simulink model "Racing_2019"  (R2017a)
settings: Solver=FixedStepDiscrete  StartTime=0.0  StopTime=Inf  FixedStep=1e-3  RelTol=1e-3  EnableMultiTasking=on
PostLoadFcn:
  | , if any(exist('dsrtsu_mdlpostloadfcn', 'file') == [2, 3, 6]), try dsrtsu_mdlpostloadfcn('Execute', bdroot); catch fprintf('Error in PostLoadFcn (dsrtsu_mdlpostloadfcn) for model "%s":\n %s\n', bdroot, lasterr); end, end,
undefined symbols (not defined in the file): Accu_Fans_Enable, Accu_Fans_ON, Accu_Fans_PWM, APPS_Bypass, APPS_Value, AUX_Error_Time, Batt_Temp_High_Threshold, Batt_Temp_Low_Threshold, BMS_Error_Time, BMS_Reset, BMS_Reset_Enable, BMS_Status_Bypass, Brake_Plausibility_Threshold, Brake_Threshold, Brakelight_Test, Braking_Torque, BSPD_State_Bypass, Buzzer, Buzzer_Silent, Buzzer_Test, Calibrate, CAN_Rx_FMEA_Enable, CAN_Status_FMEA_Enable, CAN_Tx_FMEA_Enable, Car_Reset, Car_Reset_Enable, Dash_Fan_PWM, DiscIntNeverNeededParam, DRS_Enable, DRS_PWM_OFF, DRS_PWM_ON, ED_Enable, ED_On, Eject_USB, Enable_Kill, Enable_LED_Test, Fans_Left_Enable, Fans_Left_ON, Fans_Left_PWM, Fans_Right_Enable, Fans_Right_ON, Fans_Right_PWM, I_MAX, IGBT_Temp_High_Threshold, IGBT_Temp_Low_Threshold, Inverter_CAN_Tx_Enable, Inverter_Frequency, KW_Max_Regen_Reset, KW_Max_Reset, LV_DCDC_Temp_High_Threshold, LV_DCDC_Temp_Low_Threshold, magnitude, Plausibility_Bypass, Power_Limiter_Killswitch, Power_Target_kW, Pump_Left_Enable, Pump_Left_ON, Pump_Right_Enable, Pump_Right_ON, Pump_Signal_Left ... (+13)
libraries: rtiusbflightreclib x206, simulink x153, rtican x52, powerlib_meascontrol x47, simulink_extras x17, rti1401lib_adc_type4 x6, rti1401lib_dio_type4 x3, rti1401lib_II_base x1
(part 22 of 23)

== system Racing_2019/CAN Configuration/Accu CAN Rx ==
  Rx Messages : Inport
  Accu Baudrate Rx : Memory  InheritSampleTime=on
  Compare To Constant : simulink/Logic and Bit Operations/Compare To Constant  relop=>=  const=999  OutDataTypeStr=boolean
  Counter Limited : simulink/Sources/Counter Limited  uplimit=1000  tsamp=0.001
  Delay 2ms : Delay
  Memory1 : Memory  InheritSampleTime=on
  Moving Baudrate : Sum  Inputs=+-
  Switch : Switch  Criteria=u2 > Threshold
  Switch1 : Switch  Criteria=u2 > Threshold
  "Rx Baudrate " : Outport
  wires:
  Switch/1 -> Memory1/1
  Memory1/1 -> Moving Baudrate/2, Switch/3
  Counter Limited/1 -> Compare To Constant/1
  Switch1/1 -> Accu Baudrate Rx/1
  Compare To Constant/1 -> Delay 2ms/1, Switch1/2
  Accu Baudrate Rx/1 -> "Rx Baudrate "/1, Switch1/3
  Delay 2ms/1 -> Switch/2
  Rx Messages/1 -> Moving Baudrate/1, Switch/1
  Moving Baudrate/1 -> Switch1/1

== system Racing_2019/CAN Configuration/Accu CAN Tx ==
  Tx Messages : Inport
  Accu Baudrate Tx : Memory  InheritSampleTime=on
  Compare To Constant : simulink/Logic and Bit Operations/Compare To Constant  relop=>=  const=999  OutDataTypeStr=boolean
  Counter Limited : simulink/Sources/Counter Limited  uplimit=1000  tsamp=0.001
  Delay 2ms : Delay
  Memory1 : Memory  InheritSampleTime=on
  Moving Baudrate : Sum  Inputs=+-
  Switch : Switch  Criteria=u2 > Threshold
  Switch1 : Switch  Criteria=u2 > Threshold
  "Tx Baudrate " : Outport
  wires:
  Switch/1 -> Memory1/1
  Memory1/1 -> Moving Baudrate/2, Switch/3
  Counter Limited/1 -> Compare To Constant/1
  Switch1/1 -> Accu Baudrate Tx/1
  Compare To Constant/1 -> Delay 2ms/1, Switch1/2
  Accu Baudrate Tx/1 -> "Tx Baudrate "/1, Switch1/3
  Delay 2ms/1 -> Switch/2
  Tx Messages/1 -> Moving Baudrate/1, Switch/1
  Moving Baudrate/1 -> Switch1/1

== system Racing_2019/CAN Configuration/Dash-Aux CAN Rx ==
  Rx Messages : Inport
  Compare To Constant : simulink/Logic and Bit Operations/Compare To Constant  relop=>=  const=999  OutDataTypeStr=boolean
  Counter Limited : simulink/Sources/Counter Limited  uplimit=1000  tsamp=0.001
  Dash-Aux Baudrate Rx : Memory  InheritSampleTime=on
  Delay 2ms : Delay
  Memory1 : Memory  InheritSampleTime=on
  Moving Baudrate : Sum  Inputs=+-
  Switch : Switch  Criteria=u2 > Threshold
  Switch1 : Switch  Criteria=u2 > Threshold
  Rx Baudrate : Outport
  wires:
  Switch/1 -> Memory1/1
  Memory1/1 -> Moving Baudrate/2, Switch/3
  Counter Limited/1 -> Compare To Constant/1
  Switch1/1 -> Dash-Aux Baudrate Rx/1
  Compare To Constant/1 -> Delay 2ms/1, Switch1/2
  Dash-Aux Baudrate Rx/1 -> Rx Baudrate/1, Switch1/3
  Delay 2ms/1 -> Switch/2
  Rx Messages/1 -> Moving Baudrate/1, Switch/1
  Moving Baudrate/1 -> Switch1/1

== system Racing_2019/CAN Configuration/Dash-Aux CAN Tx ==
  Tx Messages : Inport
  Compare To Constant : simulink/Logic and Bit Operations/Compare To Constant  relop=>=  const=999  OutDataTypeStr=boolean
  Counter Limited : simulink/Sources/Counter Limited  uplimit=1000  tsamp=0.001
  Dash-Aux Baudrate Tx : Memory  InheritSampleTime=on
  Delay 2ms : Delay
  Memory1 : Memory  InheritSampleTime=on
  Moving Baudrate : Sum  Inputs=+-
  Switch : Switch  Criteria=u2 > Threshold
  Switch1 : Switch  Criteria=u2 > Threshold
  Tx Baudrate : Outport
  wires:
  Switch/1 -> Memory1/1
  Memory1/1 -> Moving Baudrate/2, Switch/3
  Counter Limited/1 -> Compare To Constant/1
  Switch1/1 -> Dash-Aux Baudrate Tx/1
  Compare To Constant/1 -> Delay 2ms/1, Switch1/2
  Dash-Aux Baudrate Tx/1 -> Tx Baudrate/1, Switch1/3
  Delay 2ms/1 -> Switch/2
  Tx Messages/1 -> Moving Baudrate/1, Switch/1
  Moving Baudrate/1 -> Switch1/1

== system Racing_2019/CAN Configuration/Inverter LEFT CAN Rx ==
  Rx Messages : Inport
  Compare To Constant : simulink/Logic and Bit Operations/Compare To Constant  relop=>=  const=999  OutDataTypeStr=boolean
  Counter Limited : simulink/Sources/Counter Limited  uplimit=1000  tsamp=0.001
  Delay 2ms : Delay
  Inverter LEFT Baudrate Rx : Memory  InheritSampleTime=on
  Memory1 : Memory  InheritSampleTime=on
  Moving Baudrate : Sum  Inputs=+-
  Switch : Switch  Criteria=u2 > Threshold
  Switch1 : Switch  Criteria=u2 > Threshold
  "Rx Baudrate " : Outport
  wires:
  Switch/1 -> Memory1/1
  Memory1/1 -> Moving Baudrate/2, Switch/3
  Counter Limited/1 -> Compare To Constant/1
  Switch1/1 -> Inverter LEFT Baudrate Rx/1
  Compare To Constant/1 -> Delay 2ms/1, Switch1/2
  Inverter LEFT Baudrate Rx/1 -> "Rx Baudrate "/1, Switch1/3
  Delay 2ms/1 -> Switch/2
  Rx Messages/1 -> Moving Baudrate/1, Switch/1
  Moving Baudrate/1 -> Switch1/1

== system Racing_2019/CAN Configuration/Inverter LEFT CAN Tx ==
  Tx Messages : Inport
  Compare To Constant : simulink/Logic and Bit Operations/Compare To Constant  relop=>=  const=999  OutDataTypeStr=boolean
  Counter Limited : simulink/Sources/Counter Limited  uplimit=1000  tsamp=0.001
  Delay 2ms : Delay
  Inverter LEFT Baudrate Tx : Memory  InheritSampleTime=on
  Memory1 : Memory  InheritSampleTime=on
  Moving Baudrate : Sum  Inputs=+-
  Switch : Switch  Criteria=u2 > Threshold
  Switch1 : Switch  Criteria=u2 > Threshold
  Tx Baudrate : Outport
  wires:
  Switch/1 -> Memory1/1
  Memory1/1 -> Moving Baudrate/2, Switch/3
  Counter Limited/1 -> Compare To Constant/1
  Switch1/1 -> Inverter LEFT Baudrate Tx/1
  Compare To Constant/1 -> Delay 2ms/1, Switch1/2
  Inverter LEFT Baudrate Tx/1 -> Tx Baudrate/1, Switch1/3
  Delay 2ms/1 -> Switch/2
  Tx Messages/1 -> Moving Baudrate/1, Switch/1
  Moving Baudrate/1 -> Switch1/1

== system Racing_2019/CAN Configuration/Inverter RIGHT CAN Rx ==
  Rx Messages : Inport
  Compare To Constant : simulink/Logic and Bit Operations/Compare To Constant  relop=>=  const=999  OutDataTypeStr=boolean
  Counter Limited : simulink/Sources/Counter Limited  uplimit=1000  tsamp=0.001
  Delay 1ms : Delay  DelayLength=1
  Inverter RIGHT Baudrate Rx : Memory  InheritSampleTime=on
  Memory1 : Memory  InheritSampleTime=on
  Moving Baudrate : Sum  Inputs=+-
  Switch : Switch  Criteria=u2 > Threshold
  Switch1 : Switch  Criteria=u2 > Threshold
  "Rx Baudrate " : Outport
  wires:
  Switch/1 -> Memory1/1
  Memory1/1 -> Moving Baudrate/2, Switch/3
  Counter Limited/1 -> Compare To Constant/1
  Switch1/1 -> Inverter RIGHT Baudrate Rx/1
  Compare To Constant/1 -> Delay 1ms/1, Switch1/2
  Inverter RIGHT Baudrate Rx/1 -> "Rx Baudrate "/1, Switch1/3
  Delay 1ms/1 -> Switch/2
  Rx Messages/1 -> Moving Baudrate/1, Switch/1
  Moving Baudrate/1 -> Switch1/1

== system Racing_2019/CAN Configuration/Inverter RIGHT CAN Tx ==
  Tx Messages : Inport
  Compare To Constant : simulink/Logic and Bit Operations/Compare To Constant  relop=>=  const=999  OutDataTypeStr=boolean
  Counter Limited : simulink/Sources/Counter Limited  uplimit=1000  tsamp=0.001
  Delay 1ms : Delay  DelayLength=1
  Inverter LEFT Baudrate Tx : Memory  InheritSampleTime=on
  Memory1 : Memory  InheritSampleTime=on
  Moving Baudrate : Sum  Inputs=+-
  Switch : Switch  Criteria=u2 > Threshold
  Switch1 : Switch  Criteria=u2 > Threshold
  "Tx Baudrate " : Outport
  wires:
  Switch/1 -> Memory1/1
  Memory1/1 -> Moving Baudrate/2, Switch/3
  Counter Limited/1 -> Compare To Constant/1
  Switch1/1 -> Inverter LEFT Baudrate Tx/1
  Compare To Constant/1 -> Delay 1ms/1, Switch1/2
  Inverter LEFT Baudrate Tx/1 -> "Tx Baudrate "/1, Switch1/3
  Delay 1ms/1 -> Switch/2
  Tx Messages/1 -> Moving Baudrate/1, Switch/1
  Moving Baudrate/1 -> Switch1/1

== system Racing_2019/General Inputs/Dynamic Offset LEM IAC Left  ==
  Value : Inport
  Add : Sum
  Average Offset LEM Left : Product  Inputs=*/
  Compare To Constant : simulink/Logic and Bit Operations/Compare To Constant  relop=>=  const=10000  OutDataTypeStr=boolean
  Compare To Constant1 : simulink/Logic and Bit Operations/Compare To Constant  relop=<=  const=10001  OutDataTypeStr=boolean
  Constant : Constant  Value=0
  Constant1 : Constant  Value=Calibrate
  Constant2 : Constant  Value=0
  Counter Free-Running : simulink/Sources/Counter Free-Running  NumBits=14  tsamp=-1
  Delay : Delay  DelayLength=1
  Dynamic Offset LEM Left : Memory  InheritSampleTime=on
  Logical Operator : Logic  Operator=OR  AllPortsSameDT=off  OutDataTypeStr=boolean
  Logical Operator1 : Logic  Operator=NOT  AllPortsSameDT=off  OutDataTypeStr=boolean
  Logical Operator2 : Logic  AllPortsSameDT=off  OutDataTypeStr=boolean
  Memory LEM IAC Left : Memory
  S-R Flip-Flop LEM Left : simulink_extras/Flip Flops/S-R Flip-Flop  initial_condition=0
  Switch : Switch  Criteria=u2 > Threshold
  Switch1 : Switch  Criteria=u2 > Threshold
  Terminator : Terminator
  LEM IAC Left Dynamic Offset : Outport
  wires:
  Counter Free-Running/1 -> Compare To Constant/1, Average Offset LEM Left/2, Compare To Constant1/1
  Switch/1 -> Dynamic Offset LEM Left/1
  Memory LEM IAC Left/1 -> Average Offset LEM Left/1, Add/1
  Dynamic Offset LEM Left/1 -> LEM IAC Left Dynamic Offset/1, Switch/1
  Value/1 -> Add/2
  Average Offset LEM Left/1 -> Switch/3
  S-R Flip-Flop LEM Left/1 -> Switch/2
  S-R Flip-Flop LEM Left/2 -> Terminator/1
  Constant/1 -> Logical Operator/1
  Logical Operator/1 -> S-R Flip-Flop LEM Left/2
  Constant1/1 -> Logical Operator/2
  Switch1/1 -> Memory LEM IAC Left/1
  Add/1 -> Switch1/1
  Constant2/1 -> Switch1/3
  Logical Operator1/1 -> Delay/1
  Delay/1 -> Switch1/2
  Logical Operator2/1 -> S-R Flip-Flop LEM Left/1
  Compare To Constant/1 -> Logical Operator1/1, Logical Operator2/1
  Compare To Constant1/1 -> Logical Operator2/2

== system Racing_2019/General Inputs/Dynamic Offset LEM IAC Right ==
  Value : Inport
  Add : Sum
  Average Offset LEM Right : Product  Inputs=*/
  Compare To Constant : simulink/Logic and Bit Operations/Compare To Constant  relop=>=  const=10000  OutDataTypeStr=boolean
  Compare To Constant1 : simulink/Logic and Bit Operations/Compare To Constant  relop=<=  const=10001  OutDataTypeStr=boolean
  Constant : Constant  Value=0
  Constant1 : Constant  Value=Calibrate
  Constant2 : Constant  Value=0
  Counter Free-Running : simulink/Sources/Counter Free-Running  NumBits=14  tsamp=-1
  Delay : Delay  DelayLength=1
  Dynamic Offset LEM Right : Memory  InheritSampleTime=on
  Logical Operator : Logic  Operator=OR  AllPortsSameDT=off  OutDataTypeStr=boolean
  Logical Operator1 : Logic  Operator=NOT  AllPortsSameDT=off  OutDataTypeStr=boolean
  Logical Operator2 : Logic  AllPortsSameDT=off  OutDataTypeStr=boolean
  Memory LEM IAC Right : Memory
  S-R Flip-Flop LEM Right : simulink_extras/Flip Flops/S-R Flip-Flop  initial_condition=0
  Switch : Switch  Criteria=u2 > Threshold
  Switch1 : Switch  Criteria=u2 > Threshold
  Terminator : Terminator
  LEM IAC Right Dynamic Offset : Outport
  wires:
  Counter Free-Running/1 -> Compare To Constant/1, Average Offset LEM Right/2, Compare To Constant1/1
  Switch/1 -> Dynamic Offset LEM Right/1
  Memory LEM IAC Right/1 -> Average Offset LEM Right/1, Add/1
  Dynamic Offset LEM Right/1 -> LEM IAC Right Dynamic Offset/1, Switch/1
  Value/1 -> Add/2
  Average Offset LEM Right/1 -> Switch/3
  S-R Flip-Flop LEM Right/1 -> Switch/2
  S-R Flip-Flop LEM Right/2 -> Terminator/1
  Constant/1 -> Logical Operator/1
  Logical Operator/1 -> S-R Flip-Flop LEM Right/2
  Constant1/1 -> Logical Operator/2
  Switch1/1 -> Memory LEM IAC Right/1
  Add/1 -> Switch1/1
  Constant2/1 -> Switch1/3
  Logical Operator1/1 -> Delay/1
  Delay/1 -> Switch1/2
  Logical Operator2/1 -> S-R Flip-Flop LEM Right/1
  Compare To Constant/1 -> Logical Operator1/1, Logical Operator2/1
  Compare To Constant1/1 -> Logical Operator2/2

== system Racing_2019/General Inputs/Dynamic Offset LEM IDC ==
  Value : Inport
  Add : Sum
  Average Offset LEM IDC : Product  Inputs=*/
  Compare To Constant : simulink/Logic and Bit Operations/Compare To Constant  relop=>=  const=10000  OutDataTypeStr=boolean
  Compare To Constant1 : simulink/Logic and Bit Operations/Compare To Constant  relop=<=  const=10001  OutDataTypeStr=boolean
  Constant : Constant  Value=0
  Constant1 : Constant  Value=Calibrate
  Constant2 : Constant  Value=0
  Counter Free-Running : simulink/Sources/Counter Free-Running  NumBits=14  tsamp=-1
  Delay : Delay  DelayLength=1
  Dynamic Offset LEM IDC : Memory  InheritSampleTime=on
  Logical Operator : Logic  Operator=OR  AllPortsSameDT=off  OutDataTypeStr=boolean
  Logical Operator1 : Logic  Operator=NOT  AllPortsSameDT=off  OutDataTypeStr=boolean
  Logical Operator2 : Logic  AllPortsSameDT=off  OutDataTypeStr=boolean
  Memory LEM IDC : Memory
  S-R Flip-Flop LEM IDC : simulink_extras/Flip Flops/S-R Flip-Flop  initial_condition=0
  Switch : Switch  Criteria=u2 > Threshold
  Switch1 : Switch  Criteria=u2 > Threshold
  Terminator : Terminator
  LEM IDC Dynamic Offset : Outport
  wires:
  Counter Free-Running/1 -> Compare To Constant/1, Average Offset LEM IDC/2, Compare To Constant1/1
  Switch/1 -> Dynamic Offset LEM IDC/1
  Memory LEM IDC/1 -> Average Offset LEM IDC/1, Add/1
  Dynamic Offset LEM IDC/1 -> LEM IDC Dynamic Offset/1, Switch/1
  Value/1 -> Add/2
  Average Offset LEM IDC/1 -> Switch/3
  S-R Flip-Flop LEM IDC/1 -> Switch/2
  S-R Flip-Flop LEM IDC/2 -> Terminator/1
  Constant/1 -> Logical Operator/1
  Logical Operator/1 -> S-R Flip-Flop LEM IDC/2
  Constant1/1 -> Logical Operator/2
  Switch1/1 -> Memory LEM IDC/1
  Add/1 -> Switch1/1
  Constant2/1 -> Switch1/3
  Logical Operator1/1 -> Delay/1
  Delay/1 -> Switch1/2
  Logical Operator2/1 -> S-R Flip-Flop LEM IDC/1
  Compare To Constant/1 -> Logical Operator1/1, Logical Operator2/1
  Compare To Constant1/1 -> Logical Operator2/2

== system Racing_2019/General Inputs/Dynamic Offset LEM VDC ==
  Value : Inport
  Add : Sum
  Average Offset LEM VDC : Product  Inputs=*/
  Compare To Constant : simulink/Logic and Bit Operations/Compare To Constant  relop=>=  const=10000  OutDataTypeStr=boolean
  Compare To Constant1 : simulink/Logic and Bit Operations/Compare To Constant  relop=<=  const=10001  OutDataTypeStr=boolean
  Constant : Constant  Value=0
  Constant1 : Constant  Value=Calibrate
  Constant2 : Constant  Value=0
  Counter Free-Running : simulink/Sources/Counter Free-Running  NumBits=14  tsamp=-1
  Delay : Delay  DelayLength=1
  Dynamic Offset LEM VDC : Memory  InheritSampleTime=on
  Logical Operator : Logic  Operator=OR  AllPortsSameDT=off  OutDataTypeStr=boolean
  Logical Operator1 : Logic  Operator=NOT  AllPortsSameDT=off  OutDataTypeStr=boolean
  Logical Operator2 : Logic  AllPortsSameDT=off  OutDataTypeStr=boolean
  Memory LEM VDC : Memory
  S-R Flip-Flop LEM VDC : simulink_extras/Flip Flops/S-R Flip-Flop  initial_condition=0
  Switch : Switch  Criteria=u2 > Threshold
  Switch1 : Switch  Criteria=u2 > Threshold
  Terminator : Terminator
  LEM IAC VDC Dynamic Offset : Outport
  wires:
  Counter Free-Running/1 -> Compare To Constant/1, Average Offset LEM VDC/2, Compare To Constant1/1
  Switch/1 -> Dynamic Offset LEM VDC/1
  Memory LEM VDC/1 -> Average Offset LEM VDC/1, Add/1
  Dynamic Offset LEM VDC/1 -> LEM IAC VDC Dynamic Offset/1, Switch/1
  Value/1 -> Add/2
  Average Offset LEM VDC/1 -> Switch/3
  S-R Flip-Flop LEM VDC/1 -> Switch/2
  S-R Flip-Flop LEM VDC/2 -> Terminator/1
  Constant/1 -> Logical Operator/1
  Logical Operator/1 -> S-R Flip-Flop LEM VDC/2
  Constant1/1 -> Logical Operator/2
  Switch1/1 -> Memory LEM VDC/1
  Add/1 -> Switch1/1
  Constant2/1 -> Switch1/3
  Logical Operator1/1 -> Delay/1
  Delay/1 -> Switch1/2
  Logical Operator2/1 -> S-R Flip-Flop LEM VDC/1
  Compare To Constant/1 -> Logical Operator1/1, Logical Operator2/1
  Compare To Constant1/1 -> Logical Operator2/2

== system Racing_2019/Inverter LEFT CAN Rx/Air Temp LEFT Raw ==
  In1 : Inport
  Action Port : ActionPort  ActionType=case
  Out1 : Outport
  wires:
  In1/1 -> Out1/1

== system Racing_2019/Inverter LEFT CAN Rx/BTB LEFT Raw ==
  In1 : Inport
  Action Port : ActionPort  ActionType=case
  Out1 : Outport
  wires:
  In1/1 -> Out1/1

== system Racing_2019/Inverter LEFT CAN Rx/Commanded Torque LEFT ==
  In1 : Inport
  Action Port : ActionPort  ActionType=case
  Out1 : Outport
  wires:
  In1/1 -> Out1/1

== system Racing_2019/Inverter LEFT CAN Rx/Error LEFT Raw ==
  In1 : Inport
  Action Port : ActionPort  ActionType=case
  Out1 : Outport
  wires:
  In1/1 -> Out1/1

== system Racing_2019/Inverter LEFT CAN Rx/IGBT Temp LEFT Raw ==
  In1 : Inport
  Action Port : ActionPort  ActionType=case
  Out1 : Outport
  wires:
  In1/1 -> Out1/1

== system Racing_2019/Inverter LEFT CAN Rx/Icont LEFT Raw  ==
  In1 : Inport
  Action Port : ActionPort  ActionType=case
  Out1 : Outport
  wires:
  In1/1 -> Out1/1

== system Racing_2019/Inverter LEFT CAN Rx/Ipeak LEFT Raw ==
  In1 : Inport
  Action Port : ActionPort  ActionType=case
  Out1 : Outport
  wires:
  In1/1 -> Out1/1

== system Racing_2019/Inverter LEFT CAN Rx/Irms LEFT Raw ==
  In1 : Inport
  Action Port : ActionPort  ActionType=case
  Out1 : Outport
  wires:
  In1/1 -> Out1/1

== system Racing_2019/Inverter LEFT CAN Rx/Motor Power LEFT Raw ==
  In1 : Inport
  Action Port : ActionPort  ActionType=case
  Out1 : Outport
  wires:
  In1/1 -> Out1/1

== system Racing_2019/Inverter LEFT CAN Rx/Motor Temp LEFT Raw ==
  In1 : Inport
  Action Port : ActionPort  ActionType=case
  Out1 : Outport
  wires:
  In1/1 -> Out1/1

== system Racing_2019/Inverter LEFT CAN Rx/RPM LEFT Raw  ==
  In1 : Inport
  Action Port : ActionPort  ActionType=case
  Out1 : Outport
  wires:
  In1/1 -> Out1/1

== system Racing_2019/Inverter LEFT CAN Rx/RPM Limit LEFT Raw ==
  In1 : Inport
  Action Port : ActionPort  ActionType=case
  Out1 : Outport
  wires:
  In1/1 -> Out1/1

== system Racing_2019/Inverter LEFT CAN Rx/Vout LEFT ==
  In1 : Inport
  Action Port : ActionPort  ActionType=case
  Out1 : Outport
  wires:
  In1/1 -> Out1/1

== system Racing_2019/Inverter RIGHT CAN Rx/Air Temp RIGHT Raw ==
  In1 : Inport
  Action Port : ActionPort  ActionType=case
  Out1 : Outport
  wires:
  In1/1 -> Out1/1

== system Racing_2019/Inverter RIGHT CAN Rx/BTB RIGHT Raw ==
  In1 : Inport
  Action Port : ActionPort  ActionType=case
  Out1 : Outport
  wires:
  In1/1 -> Out1/1

== system Racing_2019/Inverter RIGHT CAN Rx/Command Torque RIGHT ==
  In1 : Inport
  Action Port : ActionPort  ActionType=case
  Out1 : Outport
  wires:
  In1/1 -> Out1/1

== system Racing_2019/Inverter RIGHT CAN Rx/Error RIGHT Raw ==
  In1 : Inport
  Action Port : ActionPort  ActionType=case
  Out1 : Outport
  wires:
  In1/1 -> Out1/1

== system Racing_2019/Inverter RIGHT CAN Rx/IGBT Temp RIGHT Raw ==
  In1 : Inport
  Action Port : ActionPort  ActionType=case
  Out1 : Outport
  wires:
  In1/1 -> Out1/1

== system Racing_2019/Inverter RIGHT CAN Rx/Icont RIGHT Raw  ==
  In1 : Inport
  Action Port : ActionPort  ActionType=case
  Out1 : Outport
  wires:
  In1/1 -> Out1/1

== system Racing_2019/Inverter RIGHT CAN Rx/Ipeak RIGHT Raw ==
  In1 : Inport
  Action Port : ActionPort  ActionType=case
  Out1 : Outport
  wires:
  In1/1 -> Out1/1

== system Racing_2019/Inverter RIGHT CAN Rx/Irms RIGHT Raw ==
  In1 : Inport
  Action Port : ActionPort  ActionType=case
  Out1 : Outport
  wires:
  In1/1 -> Out1/1

== system Racing_2019/Inverter RIGHT CAN Rx/Motor Power RIGHT Raw ==
  In1 : Inport
  Action Port : ActionPort  ActionType=case
  Out1 : Outport
  wires:
  In1/1 -> Out1/1

== system Racing_2019/Inverter RIGHT CAN Rx/Motor Temp RIGHT Raw ==
  In1 : Inport
  Action Port : ActionPort  ActionType=case
  Out1 : Outport
  wires:
  In1/1 -> Out1/1

== system Racing_2019/Inverter RIGHT CAN Rx/RPM Limit RIGHT Raw ==
  In1 : Inport
  Action Port : ActionPort  ActionType=case
  Out1 : Outport
  wires:
  In1/1 -> Out1/1

== system Racing_2019/Inverter RIGHT CAN Rx/RPM RIGHT Raw  ==
  In1 : Inport
  Action Port : ActionPort  ActionType=case
  Out1 : Outport
  wires:
  In1/1 -> Out1/1

== system Racing_2019/Inverter RIGHT CAN Rx/Vout RIGHT Raw ==
  In1 : Inport
  Action Port : ActionPort  ActionType=case
  Out1 : Outport
  wires:
  In1/1 -> Out1/1

== system Racing_2019/RTI Data/RTI Data Store ==
  RTI Data Store : Subsystem  mask(RTI_DATA_STORE){}
      mask help:
      | RTI Data Store Block. This block is used by RTI to store internal model dependent data. Deleting this block will result in data loss.
      |
      | NEVER DELETE, COPY, OR MODIFY THIS BLOCK!
      mask Help:
      | RTI Data Store Block. This block is used by RTI to store internal model dependent data. Deleting this block will result in data loss.
      | 
      | NEVER DELETE, COPY, OR MODIFY THIS BLOCK!
      mask Display: text(0.5, 0.5, ' ', 'HorizontalAlignment', 'center');

== system Racing_2019/Sensor Error Check/Counter ==
  In1 : Inport
  Add5 : Sum
  Brake_Error_Counter : Memory  InheritSampleTime=on
  Data Type Conversion13 : DataTypeConversion  OutDataTypeStr=uint8
  Edge Detector4 : powerlib_meascontrol/Logic/Edge Detector  model=Rising  ic=0  Ts=-1
      settings: SourceProductName=Simscape Power Systems  SourceProductBaseCode=PS
  wires:
  Brake_Error_Counter/1 -> Add5/2
  Add5/1 -> Brake_Error_Counter/1
  Data Type Conversion13/1 -> Add5/1
  Edge Detector4/1 -> Data Type Conversion13/1
  In1/1 -> Edge Detector4/1

== system Racing_2019/Sensor Error Check/Counter1 ==
  In1 : Inport
  APPS1_Error_Counter : Memory  InheritSampleTime=on
  Add5 : Sum
  Data Type Conversion13 : DataTypeConversion  OutDataTypeStr=uint8
  Edge Detector4 : powerlib_meascontrol/Logic/Edge Detector  model=Rising  ic=0  Ts=-1
      settings: SourceProductName=Simscape Power Systems  SourceProductBaseCode=PS
  wires:
  APPS1_Error_Counter/1 -> Add5/2
  Add5/1 -> APPS1_Error_Counter/1
  Data Type Conversion13/1 -> Add5/1
  Edge Detector4/1 -> Data Type Conversion13/1
  In1/1 -> Edge Detector4/1

== system Racing_2019/Sensor Error Check/Counter2 ==
  In1 : Inport
  APPS_NotAgree_Error_Counter : Memory  InheritSampleTime=on
  Add5 : Sum
  Data Type Conversion13 : DataTypeConversion  OutDataTypeStr=uint8
  Edge Detector4 : powerlib_meascontrol/Logic/Edge Detector  model=Rising  ic=0  Ts=-1
      settings: SourceProductName=Simscape Power Systems  SourceProductBaseCode=PS
  wires:
  APPS_NotAgree_Error_Counter/1 -> Add5/2
  Add5/1 -> APPS_NotAgree_Error_Counter/1
  Data Type Conversion13/1 -> Add5/1
  Edge Detector4/1 -> Data Type Conversion13/1
  In1/1 -> Edge Detector4/1

== system Racing_2019/Sensor Error Check/Counter3 ==
  In1 : Inport
  APPS2_Error_Counter : Memory  InheritSampleTime=on
  Add5 : Sum
  Data Type Conversion13 : DataTypeConversion  OutDataTypeStr=uint8
  Edge Detector4 : powerlib_meascontrol/Logic/Edge Detector  model=Rising  ic=0  Ts=-1
      settings: SourceProductName=Simscape Power Systems  SourceProductBaseCode=PS
  wires:
  APPS2_Error_Counter/1 -> Add5/2
  Add5/1 -> APPS2_Error_Counter/1
  Data Type Conversion13/1 -> Add5/1
  Edge Detector4/1 -> Data Type Conversion13/1
  In1/1 -> Edge Detector4/1

== system Racing_2019/Sensor Error Check/Counter4 ==
  In1 : Inport
  Add5 : Sum
  Data Type Conversion13 : DataTypeConversion  OutDataTypeStr=uint8
  Edge Detector4 : powerlib_meascontrol/Logic/Edge Detector  model=Rising  ic=0  Ts=-1
      settings: SourceProductName=Simscape Power Systems  SourceProductBaseCode=PS
  Steering_Error_Counter : Memory  InheritSampleTime=on
  wires:
  Steering_Error_Counter/1 -> Add5/2
  Add5/1 -> Steering_Error_Counter/1
  Data Type Conversion13/1 -> Add5/1
  Edge Detector4/1 -> Data Type Conversion13/1
  In1/1 -> Edge Detector4/1

== system Racing_2019/Sensor Error Check/Counter5 ==
  In1 : Inport
  Add5 : Sum
  Data Type Conversion13 : DataTypeConversion  OutDataTypeStr=uint8
  Edge Detector4 : powerlib_meascontrol/Logic/Edge Detector  model=Rising  ic=0  Ts=-1
      settings: SourceProductName=Simscape Power Systems  SourceProductBaseCode=PS
  Sensor_Error_Counter : Memory  InheritSampleTime=on
  wires:
  Sensor_Error_Counter/1 -> Add5/2
  Add5/1 -> Sensor_Error_Counter/1
  Data Type Conversion13/1 -> Add5/1
  Edge Detector4/1 -> Data Type Conversion13/1
  In1/1 -> Edge Detector4/1

== system Racing_2019/The Journey of Torque/Electronic Differential ==
  Torque Right PL : Inport
  Torque Left PL : Inport  Port=2
  Steering : Inport  Port=3
  Differential Toggle : Inport  Port=4
  AddL : Sum  Inputs=+-
  AddL2 : Sum  Inputs=+-
  AddR2 : Sum  Inputs=+-
  CompareL : simulink/Logic and Bit Operations/Compare To Constant  relop=<  const=55  OutDataTypeStr=boolean
  CompareR : simulink/Logic and Bit Operations/Compare To Constant  relop=<  const=45  OutDataTypeStr=boolean
  Constant : Constant  Value=100  SampleTime=0.001
  Constant1 : Constant  Value=32  SampleTime=0.001
  Constant2 : Constant  Value=32  SampleTime=0.001
  Data Type Conversion : DataTypeConversion  OutDataTypeStr=uint8
  ED Enable : Logic  AllPortsSameDT=off  OutDataTypeStr=boolean
  ED OR : Logic  Operator=OR  AllPortsSameDT=off  OutDataTypeStr=boolean
  ED_Enable : Constant  Value=ED_Enable  VectorParams1D=off  OutDataTypeStr=uint8  SampleTime=-1
  ED_On : Constant  Value=ED_On  VectorParams1D=off  OutDataTypeStr=uint8  SampleTime=-1
  GainL2 : Gain  Gain=1/13
  GainR2 : Gain  Gain=1/13
  Product : Product
  Product1 : Product
  Rate Transition13 : RateTransition  OutPortSampleTime=1e-3
  SaturationL : Saturate  UpperLimit=1  LowerLimit=0
  SaturationR : Saturate  UpperLimit=1  LowerLimit=0
  SwitchL2 : Switch  Criteria=u2 > Threshold
  SwitchL3 : Switch  Criteria=u2 > Threshold
  SwitchR2 : Switch  Criteria=u2 > Threshold
  SwitchR3 : Switch  Criteria=u2 > Threshold
  USB_ED_Enable : rtiusbflightreclib/USB_FLIGHT_REC_BL1  VarName=ED_Enable  DataType=UInt8  SampleTime=-1  TLCFileName=rtiusbflightrecwrite  Reserved1=[]  Reserved2=[]  Reserved3=[]  Reserved4=[]  DSProperties=struct('RTI',struct('Version',uint32(3),'BlockType',struct('isSLSource',uint8(0),'isSLSink',uint8(1),'isHWSource',uint8(0),'isHWSink',uint8(0),'isSetup',uint8(0),'isInline',uint8(1),'isNonInline',uint8(0),'isInterrupt',uint8(0),'isChannelwise',uint8(0)),'IOBoardType',{{'DSUSB','FLIGHTREC'}},'UnitType','FLIGHTREC','Identifier','WRITE','DialogType','SL','BlockSet','RTIUSBFLIGHTREC','SlaveProcessor','NONE'))  RTIBlockInterface=struct('InputPortsActive',1,'InputPortsWidth',int32(1),'InputPortsDataType',{{'SS_UINT8'}},'BlockDisplay',{{['Write to\nUSB Flight Recorder'],'center'}},'IconTransparency','off','InitLevel',3,'BlockName',struct('Token',{{'USB_FLIGHT_REC_BL1'}}),'MaskDescription',['Write input to the Flight Recorder. Recorded data can be referenced by the specified variable.'],'SampleTime',{{-1}})  RTIBlockParameters=struct('VarName',{{'ED_Enable','OFF',[]}},'DataType',{{'UInt8','OFF',[]}},'SampleTime',{{-1,'OFF',[]}},'TLCFileName',{{'rtiusbflightrecwrite','OFF',[]}})  RTISFcnParameters=struct('VarName','char','DataType','char','SampleTime','double','TLCFileName','char')  RTIBlockParaDefault=struct('VarName','Var1','DataType','Single','SampleTime',-1,'TLCFileName','rtiusbflightrecwrite')
      settings: SourceProductName=dSPACE RTI USB Flight Rec Blockset
  Torque Right ED : Outport
  Torque Left ED : Outport  Port=2
  wires:
  SwitchR3/1 -> SwitchR2/1
  SwitchL3/1 -> SwitchL2/1
  Torque Right PL/1 -> SwitchL2/3, Product/1, SwitchL3/1
  Torque Left PL/1 -> SwitchR2/3, Product1/2, SwitchR3/3
  Constant/1 -> AddL/1
  SaturationL/1 -> Product/2
  SwitchL2/1 -> Torque Right ED/1
  SwitchR2/1 -> Torque Left ED/1
  AddR2/1 -> GainR2/1
  CompareL/1 -> SwitchL3/2
  Product/1 -> SwitchL3/3
  Product1/1 -> SwitchR3/1
  CompareR/1 -> SwitchR3/2
  ED_On/1 -> ED OR/2
  Differential Toggle/1 -> Rate Transition13/1
  Steering/1 -> CompareL/1, AddR2/1, AddL/2, CompareR/1
  GainR2/1 -> SaturationR/1
  Constant1/1 -> AddR2/2
  Constant2/1 -> AddL2/2
  AddL/1 -> AddL2/1
  AddL2/1 -> GainL2/1
  GainL2/1 -> SaturationL/1
  Rate Transition13/1 -> ED OR/1
  SaturationR/1 -> Product1/1
  ED OR/1 -> ED Enable/1
  ED Enable/1 -> SwitchR2/2, SwitchL2/2, Data Type Conversion/1
  ED_Enable/1 -> ED Enable/2
  Data Type Conversion/1 -> USB_ED_Enable/1

== system Racing_2019/The Journey of Torque/Power Limiter v3 (open-loop) ==
  Power Target kW : Inport
  "IDC " : Inport  Port=2
  RPM Max : Inport  Port=3
  Irms Left : Inport  Port=4
  Irms Right : Inport  Port=5
  APPS : Inport  Port=6
  12kHz : Subsystem  TreatAsAtomicUnit=on
  8kHz : Subsystem  TreatAsAtomicUnit=on
  AC Losses : Product
  AC Losses const : Constant  Value=0.0036
  APPS Killswitch : Sum
  APPS PL : Product
  Add : Sum  Inputs=-+
  "Amps " : Product  Inputs=*/
  Amps Out : simulink/Discontinuities/Saturation Dynamic  OutMin=0  OutMax=300  OutDataTypeStr=Inherit: Same as second input  OutDataType=fixdt(1, 16)  OutScaling=2^-10  DoSatur=off
  Amps Ref : Product  Inputs=*/
  Back EMF : Product
  Constant : Constant  Value=0
  DC Losses : Product
  DC Losses const : Constant  Value=0.0026
  I Max : Constant  Value=300
  "IDC Saturation " : Saturate  UpperLimit=500  LowerLimit=0
  IGBT Losses : Merge  Inputs=3  InitialOutput=500135000
  Irms Initialization : MATLAB Function  TreatAsAtomicUnit=on
  Irms Min : Switch  Criteria=u2 > Threshold
  Irms Previous : Memory
  Irms Saturation : Saturate  UpperLimit=300  LowerLimit=0
  Koimismenos : Subsystem  TreatAsAtomicUnit=on
  LUT K(t) constant : Lookup_n-D  NumberOfTableDimensions=1  BreakpointsForDimension1=[10,20,30,40,50,60,70,80,90,100,110,120,130,140,150,160,170,180,190,200,210,220,230,240,250,260,270,280,290,300]  Table=[0.709530609642927,0.716484185245995,0.720919316643401,0.724254727682334,0.726790261091103,0.728639279411534,0.729861865132176,0.730498120721597,0.730579268639483,0.730132091341083,0.72918094946104,0.727748790905312,0.72585769420836,0.723529179022966,0.720784392414125,0.717644225292734,0.714129387755025,0.710260459308867,0.706057923239121,0.701542190663395,0.69673361771472,0.691652518038047,0.686319172026786,0.680753833750209,0.674976736218279,0.669008095431517,0.662868113530898,0.656576981272769,0.650154879991719,0.643621983170869]  InternalRulePriority=Speed  RndMeth=Simplest  InputSameDT=on
  Math Function : Math  Operator=magnitude^2  SaturateOnIntegerOverflow=on
  Math Function1 : Math  Operator=magnitude^2  SaturateOnIntegerOverflow=on
  PL Disable : Constant  Value=Power_Limiter_Killswitch
  PM Gain : Gain  Gain=0.5
  Power Motors : Sum  Inputs=+---
  RPM Saturation : Saturate  UpperLimit=6000  LowerLimit=0
  RPM to rad/s : Gain  Gain=0.10479
  Switch Case : SwitchCase  CaseConditions={8,12}
  Switching Frequency : Constant  Value=Inverter_Frequency
  "Torque Limit Percentage " : Gain  Gain=100
  Torque Limiter : Saturate  UpperLimit=1  LowerLimit=0
  USB_PL_Torque_Limiter : rtiusbflightreclib/USB_FLIGHT_REC_BL1  VarName=PL_Torque_Limiter_Percentage  DataType=UInt8  SampleTime=-1  TLCFileName=rtiusbflightrecwrite  Reserved1=[]  Reserved2=[]  Reserved3=[]  Reserved4=[]  DSProperties=struct('RTI',struct('Version',uint32(3),'BlockType',struct('isSLSource',uint8(0),'isSLSink',uint8(1),'isHWSource',uint8(0),'isHWSink',uint8(0),'isSetup',uint8(0),'isInline',uint8(1),'isNonInline',uint8(0),'isInterrupt',uint8(0),'isChannelwise',uint8(0)),'IOBoardType',{{'DSUSB','FLIGHTREC'}},'UnitType','FLIGHTREC','Identifier','WRITE','DialogType','SL','BlockSet','RTIUSBFLIGHTREC','SlaveProcessor','NONE'))  RTIBlockInterface=struct('InputPortsActive',1,'InputPortsWidth',int32(1),'InputPortsDataType',{{'SS_UINT8'}},'BlockDisplay',{{['Write to\nUSB Flight Recorder'],'center'}},'IconTransparency','off','InitLevel',3,'BlockName',struct('Token',{{'USB_FLIGHT_REC_BL1'}}),'MaskDescription',['Write input to the Flight Recorder. Recorded data can be referenced by the specified variable.'],'SampleTime',{{-1}})  RTIBlockParameters=struct('VarName',{{'PL_Torque_Limiter_Percentage','OFF',[]}},'DataType',{{'UInt8','OFF',[]}},'SampleTime',{{-1,'OFF',[]}},'TLCFileName',{{'rtiusbflightrecwrite','OFF',[]}})  RTISFcnParameters=struct('VarName','char','DataType','char','SampleTime','double','TLCFileName','char')  RTIBlockParaDefault=struct('VarName','Var1','DataType','Single','SampleTime',-1,'TLCFileName','rtiusbflightrecwrite')
      settings: SourceProductName=dSPACE RTI USB Flight Rec Blockset
  Watt : Gain  Gain=1000
  conversion8 : DataTypeConversion  OutDataTypeStr=uint8
  Torque Ref PL : Outport
  wires:
  Power Target kW/1 -> Watt/1
  "IDC "/1 -> "IDC Saturation "/1
  DC Losses const/1 -> DC Losses/2
  Math Function/1 -> DC Losses/1
  RPM Max/1 -> RPM Saturation/1
  RPM Saturation/1 -> RPM to rad/s/1
  RPM to rad/s/1 -> Back EMF/1
  LUT K(t) constant/1 -> Back EMF/2
  Switching Frequency/1 -> Switch Case/1
  Switch Case/1 -> 8kHz/Action
  Switch Case/2 -> 12kHz/Action
  Switch Case/3 -> Koimismenos/Action
  Koimismenos/1(You Shall Not Run) -> IGBT Losses/3
  12kHz/1(IGBT Losses) -> IGBT Losses/2
  8kHz/1(IGBT Losses) -> IGBT Losses/1
  AC Losses const/1 -> AC Losses/2
  Math Function1/1 -> AC Losses/1
  AC Losses/1 -> Power Motors/3
  Power Motors/1 -> PM Gain/1
  Back EMF/1 -> "Amps "/2
  "Amps "/1 -> Amps Out/2
  Constant/1 -> Amps Out/3
  Irms Left/1 -> Add/1, Irms Min/1
  Irms Right/1 -> Add/2, Irms Min/3
  Add/1 -> Irms Min/2
  Amps Out/1 -> Amps Ref/1, Irms Saturation/1
  I Max/1 -> Amps Ref/2
  PL Disable/1 -> APPS Killswitch/2
  APPS Killswitch/1 -> Torque Limiter/1
  Amps Ref/1 -> APPS Killswitch/1
  APPS/1 -> APPS PL/1
  Torque Limiter/1 -> "Torque Limit Percentage "/1, APPS PL/2
  Irms Previous/1 -> Irms Initialization/1(Irms_In)
  Watt/1 -> Power Motors/1
  DC Losses/1 -> Power Motors/2
  Irms Initialization/1(Irms_Out) -> LUT K(t) constant/1, Math Function1/1, 8kHz/1(IAC Previous), 12kHz/1(IAC Previous)
  "IDC Saturation "/1 -> Math Function/1
  Irms Saturation/1 -> Irms Previous/1
  IGBT Losses/1 -> Power Motors/4
  PM Gain/1 -> "Amps "/1
  conversion8/1 -> USB_PL_Torque_Limiter/1
  "Torque Limit Percentage "/1 -> conversion8/1
  APPS PL/1 -> Torque Ref PL/1
  Irms Min/1 -> Amps Out/1

== system Racing_2019/The Journey of Torque/Regen ==
  "IDC " : Inport
  "Regen Enable " : Inport  Port=2
  Death : simulink/Logic and Bit Operations/Compare To Constant  relop=<=  const=-48  OutDataTypeStr=boolean
  IDC_Regen_last_max : simulink/Math Operations/MinMax Running Resettable  Function=min  vinit=0.0
  IDC_Regen_max : simulink/Math Operations/MinMax Running Resettable  Function=min  vinit=0.0
  Icontinuous1 : Constant  Value=Regen_IDC_Reset  OutDataTypeStr=boolean  SampleTime=-1
  Icontinuous2 : Constant  Value=Braking_Torque/4  OutDataTypeStr=uint8  SampleTime=-1
  Icontinuous5 : Constant  Value=Braking_Torque  OutDataTypeStr=uint8  SampleTime=-1
  Irms max : Constant  Value=300  SampleTime=-1
  LUT K(t) constant : Lookup_n-D  NumberOfTableDimensions=1  BreakpointsForDimension1=[10,20,30,40,50,60,70,80,90,100,110,120,130,140,150,160,170,180,190,200,210,220,230,240,250,260,270,280,290,300]  BeginIndexSearchUsingPreviousIndexResult=on  Table=[0.709530609642927,0.716484185245995,0.720919316643401,0.724254727682334,0.726790261091103,0.728639279411534,0.729861865132176,0.730498120721597,0.730579268639483,0.730132091341083,0.72918094946104,0.727748790905312,0.72585769420836,0.723529179022966,0.720784392414125,0.717644225292734,0.714129387755025,0.710260459308867,0.706057923239121,0.701542190663395,0.69673361771472,0.691652518038047,0.686319172026786,0.680753833750209,0.674976736218279,0.669008095431517,0.662868113530898,0.656576981272769,0.650154879991719,0.643621983170869]  InternalRulePriority=Speed  RndMeth=Simplest  InputSameDT=on
  Memory : Memory  InheritSampleTime=on
  RPM AND2 : Logic  Operator=NOT  AllPortsSameDT=off  OutDataTypeStr=boolean
  Rate Transition1 : RateTransition  OutPortSampleTime=1e-1
  Resettable Delay : Delay  DelayLength=1  ExternalReset=Rising
      settings: InputPortMap=u0,r5
  Switch : Switch  Criteria=u2 > Threshold
  Terminator1 : Terminator
  TorqueLeftLimiter1 : Saturate  UpperLimit=0.2  LowerLimit=0
  TorqueLeftLimiter2 : Saturate  UpperLimit=40  LowerLimit=0
  TorqueRightFiltered1 : Product  Inputs=*/  OutDataTypeStr=single
  TorqueRightFiltered2 : Product  Inputs=*/  OutDataTypeStr=single
  USB_Braking_Torque : rtiusbflightreclib/USB_FLIGHT_REC_BL1  VarName=Braking_Torque  DataType=UInt8  SampleTime=1e-1  TLCFileName=rtiusbflightrecwrite  Reserved1=[]  Reserved2=[]  Reserved3=[]  Reserved4=[]  DSProperties=struct('RTI',struct('Version',uint32(3),'BlockType',struct('isSLSource',uint8(0),'isSLSink',uint8(1),'isHWSource',uint8(0),'isHWSink',uint8(0),'isSetup',uint8(0),'isInline',uint8(1),'isNonInline',uint8(0),'isInterrupt',uint8(0),'isChannelwise',uint8(0)),'IOBoardType',{{'DSUSB','FLIGHTREC'}},'UnitType','FLIGHTREC','Identifier','WRITE','DialogType','SL','BlockSet','RTIUSBFLIGHTREC','SlaveProcessor','NONE'))  RTIBlockInterface=struct('InputPortsActive',1,'InputPortsWidth',int32(1),'InputPortsDataType',{{'SS_UINT8'}},'BlockDisplay',{{['Write to\nUSB Flight Recorder'],'center'}},'IconTransparency','off','InitLevel',3,'BlockName',struct('Token',{{'USB_FLIGHT_REC_BL1'}}),'MaskDescription',['Write input to the Flight Recorder. Recorded data can be referenced by the specified variable.'],'SampleTime',{{0.1}})  RTIBlockParameters=struct('VarName',{{'Braking_Torque','OFF',[]}},'DataType',{{'UInt8','OFF',[]}},'SampleTime',{{'1e-1','OFF',[]}},'TLCFileName',{{'rtiusbflightrecwrite','OFF',[]}})  RTISFcnParameters=struct('VarName','char','DataType','char','SampleTime','double','TLCFileName','char')  RTIBlockParaDefault=struct('VarName','Var1','DataType','Single','SampleTime',-1,'TLCFileName','rtiusbflightrecwrite')
      settings: SourceProductName=dSPACE RTI USB Flight Rec Blockset
  USB_Torque_Regen1 : rtiusbflightreclib/USB_FLIGHT_REC_BL1  VarName=Torue_before_mul  DataType=Single  SampleTime=-1  TLCFileName=rtiusbflightrecwrite  Reserved1=[]  Reserved2=[]  Reserved3=[]  Reserved4=[]  DSProperties=struct('RTI',struct('Version',uint32(3),'BlockType',struct('isSLSource',uint8(0),'isSLSink',uint8(1),'isHWSource',uint8(0),'isHWSink',uint8(0),'isSetup',uint8(0),'isInline',uint8(1),'isNonInline',uint8(0),'isInterrupt',uint8(0),'isChannelwise',uint8(0)),'IOBoardType',{{'DSUSB','FLIGHTREC'}},'UnitType','FLIGHTREC','Identifier','WRITE','DialogType','SL','BlockSet','RTIUSBFLIGHTREC','SlaveProcessor','NONE'))  RTIBlockInterface=struct('InputPortsActive',1,'InputPortsWidth',int32(1),'InputPortsDataType',{{'SS_SINGLE'}},'BlockDisplay',{{['Write to\nUSB Flight Recorder'],'center'}},'IconTransparency','off','InitLevel',3,'BlockName',struct('Token',{{'USB_FLIGHT_REC_BL1'}}),'MaskDescription',['Write input to the Flight Recorder. Recorded data can be referenced by the specified variable.'],'SampleTime',{{-1}})  RTIBlockParameters=struct('VarName',{{'Torue_before_mul','OFF',[]}},'DataType',{{'Single','OFF',[]}},'SampleTime',{{-1,'OFF',[]}},'TLCFileName',{{'rtiusbflightrecwrite','OFF',[]}})  RTISFcnParameters=struct('VarName','char','DataType','char','SampleTime','double','TLCFileName','char')  RTIBlockParaDefault=struct('VarName','Var1','DataType','Single','SampleTime',-1,'TLCFileName','rtiusbflightrecwrite')
      settings: SourceProductName=dSPACE RTI USB Flight Rec Blockset
  torGainL1 : Gain  Gain=-1000  OutDataTypeStr=double
  "Torque Ref Regen " : Outport
  wires:
  torGainL1/1 -> "Torque Ref Regen "/1
  Icontinuous1/1 -> IDC_Regen_max/2
  IDC_Regen_max/1 -> Terminator1/1
  TorqueLeftLimiter2/1 -> TorqueRightFiltered1/1, Rate Transition1/1
  TorqueLeftLimiter1/1 -> USB_Torque_Regen1/1, torGainL1/1
  Rate Transition1/1 -> USB_Braking_Torque/1
  LUT K(t) constant/1 -> TorqueRightFiltered1/2
  TorqueRightFiltered2/1 -> TorqueLeftLimiter1/1
  Irms max/1 -> TorqueRightFiltered2/2
  RPM AND2/1 -> IDC_Regen_last_max/2
  TorqueRightFiltered1/1 -> Memory/1, TorqueRightFiltered2/1
  "IDC "/1 -> Death/1, IDC_Regen_last_max/1
  "Regen Enable "/1 -> Resettable Delay/1, Resettable Delay/2
  Resettable Delay/1 -> RPM AND2/1
  Memory/1 -> LUT K(t) constant/1
  IDC_Regen_last_max/1 -> IDC_Regen_max/1
  Icontinuous5/1 -> Switch/3
  Switch/1 -> TorqueLeftLimiter2/1
  Icontinuous2/1 -> Switch/1
  Death/1 -> Switch/2

== system Racing_2019/RTI Data/RTI Data Store/RTI Data Store ==
  RTI Data Store : Subsystem  mask(RTI_DATA_STORE){}
      mask help:
      | RTI Data Store Block. This block is used by RTI to store internal model dependent data. Deleting this block will result in data loss.
      |
      | NEVER DELETE, COPY, OR MODIFY THIS BLOCK!
      mask Help:
      | RTI Data Store Block. This block is used by RTI to store internal model dependent data. Deleting this block will result in data loss.
      | 
      | NEVER DELETE, COPY, OR MODIFY THIS BLOCK!
      mask Display: text(0.5, 0.5, ' ', 'HorizontalAlignment', 'center');

== system Racing_2019/The Journey of Torque/Power Limiter v3 (open-loop)/12kHz ==
  IAC Previous : Inport
  Action Port : ActionPort  ActionType=case
  Polynomial 12kHz : Fcn  Expr=7.49434389140272e-10*u^5 - 6.63725061703005e-7*u^4 + 0.000230122634718224*u^3 - 0.0349086152817771*u^2 + 7.52169158782394*u - 25.9342657342656
  IGBT Losses : Outport
  wires:
  Polynomial 12kHz/1 -> IGBT Losses/1
  IAC Previous/1 -> Polynomial 12kHz/1

== system Racing_2019/The Journey of Torque/Power Limiter v3 (open-loop)/8kHz ==
  IAC Previous : Inport
  Action Port : ActionPort  ActionType=case
  Polynomial 8kHz : Fcn  Expr=3.59348952131459e-10*u^5 - 3.40337729221243e-07*u^4 + 0.000126380462610146*u^3 - 0.0186128468087641*u^2 + 5.60210298880688*u - 15.4523076923087
  IGBT Losses : Outport
  wires:
  Polynomial 8kHz/1 -> IGBT Losses/1
  IAC Previous/1 -> Polynomial 8kHz/1

== system Racing_2019/The Journey of Torque/Power Limiter v3 (open-loop)/Koimismenos ==
  Action Port : ActionPort  ActionType=default
  Constant : Constant  Value=500135000
  You Shall Not Run : Outport
  wires:
  Constant/1 -> You Shall Not Run/1

== system Racing_2019/RTI Data/RTI Data Store/RTI Data Store/RTI Data Store ==
  RTI Data Store : Subsystem  mask(RTI_DATA_STORE){}
      mask help:
      | RTI Data Store Block. This block is used by RTI to store internal model dependent data. Deleting this block will result in data loss.
      |
      | NEVER DELETE, COPY, OR MODIFY THIS BLOCK!
      mask Help:
      | RTI Data Store Block. This block is used by RTI to store internal model dependent data. Deleting this block will result in data loss.
      | 
      | NEVER DELETE, COPY, OR MODIFY THIS BLOCK!
      mask Display: text(0.5, 0.5, ' ', 'HorizontalAlignment', 'center');

== system Racing_2019/RTI Data/RTI Data Store/RTI Data Store/RTI Data Store/RTI Data Store ==

== matlab function Racing_2019/Accu CAN Rx/Segment 1/s1t1 ==
  data: x input; y output
function y = thermBMS(x)
y = (1/(0.003354016+0.000256524*log(((10000*x)/(5-x))/10000)+0.00000260597*(log(((10000*x)/(5-x))/100000))*(log(((10000*x)/(5-x))/10000))+0.0000000632926*(log(((100000*x)/(5-x))/10000))*(log(((10000*x)/(5-x))/10000))*(log(((10000*x)/(5-x))/10000))))-273.15
end

== matlab function Racing_2019/Accu CAN Rx/Segment 1/s1t2 ==
  data: x input; y output
function y = thermBMS(x)
y = (1/(0.003354016+0.000256524*log(((10000*x)/(5-x))/10000)+0.00000260597*(log(((10000*x)/(5-x))/100000))*(log(((10000*x)/(5-x))/10000))+0.0000000632926*(log(((100000*x)/(5-x))/10000))*(log(((10000*x)/(5-x))/10000))*(log(((10000*x)/(5-x))/10000))))-273.15
end

== matlab function Racing_2019/Accu CAN Rx/Segment 1/s1t4 ==
  data: x input; y output
function y = thermBMS(x)
y = (1/(0.003354016+0.000256524*log(((10000*x)/(5-x))/10000)+0.00000260597*(log(((10000*x)/(5-(x*0.0015)))/100000))*(log(((10000*x)/(5-x))/10000))+0.0000000632926*(log(((100000*x)/(5-x))/10000))*(log(((10000*x)/(5-x))/10000))*(log(((10000*x)/(5-x))/10000))))-273.15
end

== matlab function Racing_2019/Accu CAN Rx/Segment 1/s1t3 ==
  data: x input; y output
function y = thermBMS(x)
y = (1/(0.003354016+0.000256524*log(((10000*x)/(5-x))/10000)+0.00000260597*(log(((10000*x)/(5-x))/100000))*(log(((10000*x)/(5-x))/10000))+0.0000000632926*(log(((100000*x)/(5-x))/10000))*(log(((10000*x)/(5-x))/10000))*(log(((10000*x)/(5-x))/10000))))-273.15
end

== matlab function Racing_2019/Accu CAN Rx/Segment 2/s2t1 ==
  data: x input; y output
function y = thermBMS(x)
y = (1/(0.003354016+0.000256524*log(((10000*x)/(5-x))/10000)+0.00000260597*(log(((10000*x)/(5-x))/100000))*(log(((10000*x)/(5-x))/10000))+0.0000000632926*(log(((100000*x)/(5-x))/10000))*(log(((10000*x)/(5-x))/10000))*(log(((10000*x)/(5-x))/10000))))-273.15
end

== matlab function Racing_2019/Accu CAN Rx/Segment 2/s2t2 ==
  data: x input; y output
function y = thermBMS(x)
y = (1/(0.003354016+0.000256524*log(((10000*x)/(5-x))/10000)+0.00000260597*(log(((10000*x)/(5-x))/100000))*(log(((10000*x)/(5-x))/10000))+0.0000000632926*(log(((100000*x)/(5-x))/10000))*(log(((10000*x)/(5-x))/10000))*(log(((10000*x)/(5-x))/10000))))-273.15
end

== matlab function Racing_2019/Accu CAN Rx/Segment 2/s2t3 ==
  data: x input; y output
function y = thermBMS(x)
y = (1/(0.003354016+0.000256524*log(((10000*x)/(5-x))/10000)+0.00000260597*(log(((10000*x)/(5-x))/100000))*(log(((10000*x)/(5-x))/10000))+0.0000000632926*(log(((100000*x)/(5-x))/10000))*(log(((10000*x)/(5-x))/10000))*(log(((10000*x)/(5-x))/10000))))-273.15
end

== matlab function Racing_2019/Accu CAN Rx/Segment 2/s2t4 ==
  data: x input; y output
function y = thermBMS(x)
y = (1/(0.003354016+0.000256524*log(((10000*x)/(5-x))/10000)+0.00000260597*(log(((10000*x)/(5-(x*0.0015)))/100000))*(log(((10000*x)/(5-x))/10000))+0.0000000632926*(log(((100000*x)/(5-x))/10000))*(log(((10000*x)/(5-x))/10000))*(log(((10000*x)/(5-x))/10000))))-273.15
end

== matlab function Racing_2019/Accu CAN Rx/Segment 3/s3t1 ==
  data: x input; y output
function y = thermBMS(x)
y = (1/(0.003354016+0.000256524*log(((10000*x)/(5-x))/10000)+0.00000260597*(log(((10000*x)/(5-x))/100000))*(log(((10000*x)/(5-x))/10000))+0.0000000632926*(log(((100000*x)/(5-x))/10000))*(log(((10000*x)/(5-x))/10000))*(log(((10000*x)/(5-x))/10000))))-273.15
end

== matlab function Racing_2019/Accu CAN Rx/Segment 3/s3t2 ==
  data: x input; y output
function y = thermBMS(x)
y = (1/(0.003354016+0.000256524*log(((10000*x)/(5-x))/10000)+0.00000260597*(log(((10000*x)/(5-x))/100000))*(log(((10000*x)/(5-x))/10000))+0.0000000632926*(log(((100000*x)/(5-x))/10000))*(log(((10000*x)/(5-x))/10000))*(log(((10000*x)/(5-x))/10000))))-273.15
end

== matlab function Racing_2019/Accu CAN Rx/Segment 3/s3t3 ==
  data: x input; y output
function y = thermBMS(x)
y = (1/(0.003354016+0.000256524*log(((10000*x)/(5-x))/10000)+0.00000260597*(log(((10000*x)/(5-x))/100000))*(log(((10000*x)/(5-x))/10000))+0.0000000632926*(log(((100000*x)/(5-x))/10000))*(log(((10000*x)/(5-x))/10000))*(log(((10000*x)/(5-x))/10000))))-273.15
end

== matlab function Racing_2019/Accu CAN Rx/Segment 3/s3t4 ==
  data: x input; y output
function y = thermBMS(x)
y = (1/(0.003354016+0.000256524*log(((10000*x)/(5-x))/10000)+0.00000260597*(log(((10000*x)/(5-(x*0.0015)))/100000))*(log(((10000*x)/(5-x))/10000))+0.0000000632926*(log(((100000*x)/(5-x))/10000))*(log(((10000*x)/(5-x))/10000))*(log(((10000*x)/(5-x))/10000))))-273.15
end

== matlab function Racing_2019/Accu CAN Rx/Segment 4/s4t1 ==
  data: x input; y output
function y = thermBMS(x)
y = (1/(0.003354016+0.000256524*log(((10000*x)/(5-x))/10000)+0.00000260597*(log(((10000*x)/(5-x))/100000))*(log(((10000*x)/(5-x))/10000))+0.0000000632926*(log(((100000*x)/(5-x))/10000))*(log(((10000*x)/(5-x))/10000))*(log(((10000*x)/(5-x))/10000))))-273.15
end

== matlab function Racing_2019/Accu CAN Rx/Segment 4/s4t2 ==
  data: x input; y output
function y = thermBMS(x)
y = (1/(0.003354016+0.000256524*log(((10000*x)/(5-x))/10000)+0.00000260597*(log(((10000*x)/(5-x))/100000))*(log(((10000*x)/(5-x))/10000))+0.0000000632926*(log(((100000*x)/(5-x))/10000))*(log(((10000*x)/(5-x))/10000))*(log(((10000*x)/(5-x))/10000))))-273.15
end

== matlab function Racing_2019/Accu CAN Rx/Segment 4/s4t3 ==
  data: x input; y output
function y = thermBMS(x)
y = (1/(0.003354016+0.000256524*log(((10000*x)/(5-x))/10000)+0.00000260597*(log(((10000*x)/(5-x))/100000))*(log(((10000*x)/(5-x))/10000))+0.0000000632926*(log(((100000*x)/(5-x))/10000))*(log(((10000*x)/(5-x))/10000))*(log(((10000*x)/(5-x))/10000))))-273.15
end

== matlab function Racing_2019/Accu CAN Rx/Segment 4/s4t4 ==
  data: x input; y output
function y = thermBMS(x)
y = (1/(0.003354016+0.000256524*log(((10000*x)/(5-x))/10000)+0.00000260597*(log(((10000*x)/(5-(x*0.0015)))/100000))*(log(((10000*x)/(5-x))/10000))+0.0000000632926*(log(((100000*x)/(5-x))/10000))*(log(((10000*x)/(5-x))/10000))*(log(((10000*x)/(5-x))/10000))))-273.15
end
